simulink model "openLoop"  (Simulink 8.6)
settings: Solver=ode45  StartTime=0.0  StopTime=60  RelTol=1e-3
libraries: simulink x1, SEA_library_models x1
settings Model: Creator=joern  LastModifiedBy=wesley
settings DataIOCC: SignalLoggingSaveFormat=Dataset
settings OptimizationCC: ExpressionDepthLimit=128
settings DebuggingCC: UnderspecifiedInitializationDetection=Simplified  MergeDetectMultiDrivingBlocksExec=error  FcnCallInpInsideContextMsg=EnableAllAsError  StateNameClashWarn=none
settings GRTTargetCC: CombineOutputUpdateFcns=on  GRTInterface=off

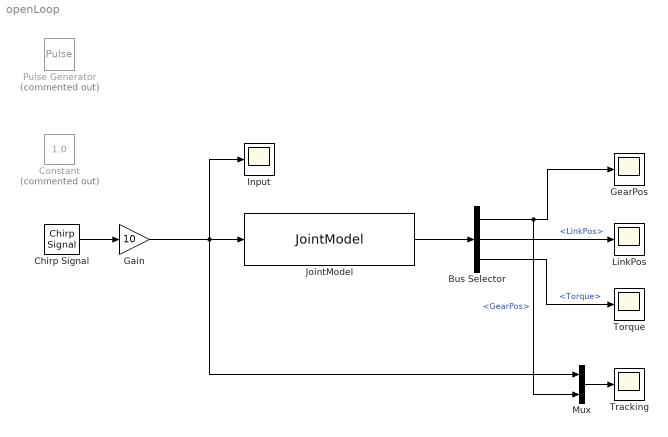
== system openLoop ==
  Bus Selector : BusSelector  OutputSignals=GearPos,LinkPos,Torque
  Chirp Signal : simulink/Sources/Chirp Signal  f1=0.1  T=60  f2=60
  Constant : Constant  Commented=on  Value=1.0
  Gain : Gain  Gain=10
  GearPos : Scope
  Input : Scope
  JointModel : SEA_library_models/Joint models/JointModel  jointObj=my_joint  fc_vel=100  fc_torque=100  input_delay=0  output_delay=0  input_noise_enabled=off  output_noise_enabled=off  var_u=0.12^2  var_y=1.8e-10
  LinkPos : Scope
  Mux : Mux  Inputs=2
  Pulse Generator : DiscretePulseGenerator  Commented=on  PulseType=Time based  Period=10  PulseWidth=0.1
  Torque : Scope
  Tracking : Scope
  wires:
  JointModel/1 -> Bus Selector/1
  Bus Selector/2 -> LinkPos/1  "<LinkPos>"
  Bus Selector/3 -> Torque/1  "<Torque>"
  Mux/1 -> Tracking/1
  Bus Selector/1 -> Mux/2, GearPos/1  "<GearPos>"
  Chirp Signal/1 -> Gain/1
  Gain/1 -> Input/1, JointModel/1, Mux/1
